simulink model "idealvehicle"  (R2020b)
settings: Solver=ode4  StartTime=0  StopTime=endtime  FixedStep=0.1  MaxStep=0.05  RelTol=1e-5
values from neighbouring files (symbols this model uses):
  Av = 2.55    [InitiateIDEAL.m]
  Cd = 0.79    [InitiateIDEAL.m]
  Cr = 0.00576    [InitiateIDEAL.m]
  Density = (85*19.6e6 + 15*32e6)/100    (= 21460000)    [InitiateIDEAL.m]
  grav = 9.81    [InitiateIDEAL.m]
  Mv = 40000    [InitiateIDEAL.m]
  Pmax = 450000    [InitiateIDEAL.m]
  rho_air = 1.2    [InitiateIDEAL.m]
  rw = 0.506    [InitiateIDEAL.m]
settings Model: ExtModeTrigMode=oneshot  ExtModeArmWhenConnect=off  Creator=Mats  LastModifiedBy=ielmats
settings DataIOCC: SaveFormat=Array  SignalLoggingSaveFormat=ModelDataLogs  ReturnWorkspaceOutputs=off  SignalLoggingName=sigsOut
settings OptimizationCC: BlockReduction=off  BooleanDataType=off  ExpressionDepthLimit=2147483647  InitFltsAndDblsToZero=on  LifeSpan=inf
settings DebuggingCC: ConsistencyChecking=warning  SaveWithParameterizedLinksMsg=none  UnderspecifiedInitializationDetection=Classic  MergeDetectMultiDrivingBlocksExec=none  SignalResolutionControl=TryResolveAllWithWarning  MultiTaskDSMMsg=warning  MultiTaskCondExecSysMsg=none  UnnecessaryDatatypeConvMsg=warning  UnconnectedInputMsg=none  UnconnectedOutputMsg=none  UnconnectedLineMsg=none  StateNameClashWarn=warning  SFUnexpectedBacktrackingDiag=warning  SFNoUnconditionalDefaultTransitionDiag=warning  ArithmeticOperatorsInVariantConditions=warning
settings HardwareCC: ProdBitPerPointer=32  ProdBitPerSizeT=32  ProdBitPerPtrDiffT=32  ProdLargestAtomicFloat=None  ProdIntDivRoundTo=Undefined  ProdEndianess=Unspecified  ProdWordSize=32  ProdHWDeviceType=32-bit Generic  TargetUnknown=on
settings ModelReferenceCC: PropagateSignalLabelsOutOfModel=off
settings SFSimCC: SimUseLocalCustomCode=off  CustomCodeUndefinedFunction=UseInterfaceOnly
settings RTWCC: RTWUseLocalCustomCode=off
settings CodeAppCC: StateflowObjectComments=on
settings GRTTargetCC: TargetLangStandard=C89/C90 (ANSI)  CombineOutputUpdateFcns=off  GRTInterface=on
settings ConfigComp: CovMetricSettings=dw  CovSaveCumulativeToWorkspaceVar=on  CovSaveSingleToWorkspaceVar=on  CovExternalEMLEnable=off

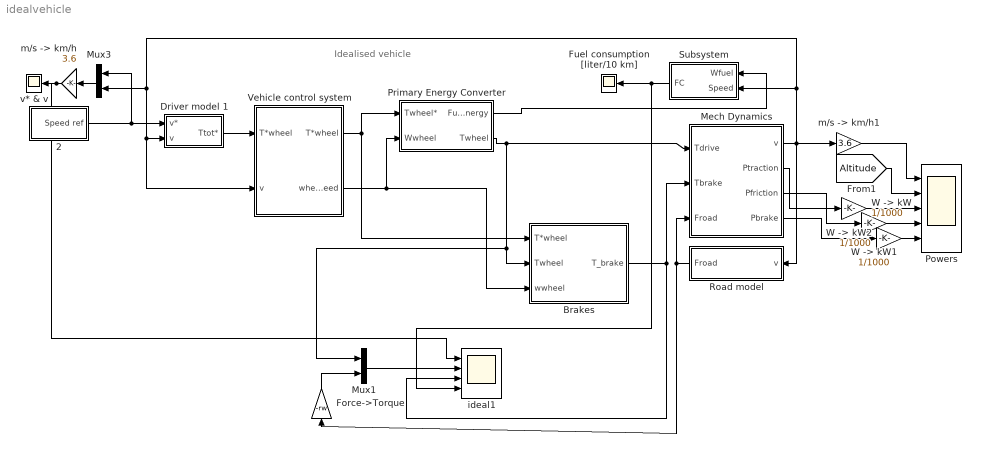
== system idealvehicle ==
  note: Idealised vehicle
  " 2" : Subsystem
  Brakes : Subsystem
  Driver model 1 : Subsystem  mask{Mv=Mv, rw=rw, Pmax=Pmax}
      mask prompts: Mv "Vehicle Mass"; rw "Wheel Radius"; Pmax "Max Wheel Power"
      mask init:
      | Ti = 2 + 1*(Mv-1000)/19000;
      | Kv=4*Mv/Ti;
  Force->Torque : Gain  Gain=-rw  SaturateOnIntegerOverflow=on  OutDataTypeStr=Inherit: Same as input  ParamDataTypeStr=Inherit: Same as input
  Fuel consumption [liter/10 km] : Scope
  Mech Dynamics : Subsystem
  Mux1 : Mux  Inputs=2
  Mux3 : Mux  Inputs=2
  Powers : Scope  NumInputPorts=5
  Primary Energy Converter : Subsystem
  Road model : Subsystem
  Subsystem : Subsystem
  Vehicle control system : Subsystem
  "W -> kW" : Gain  Gain=1/1000  SaturateOnIntegerOverflow=on  OutDataTypeStr=Inherit: Same as input  ParamDataTypeStr=Inherit: Same as input
  "W -> kW1" : Gain  Gain=1/1000  SaturateOnIntegerOverflow=on  OutDataTypeStr=Inherit: Same as input  ParamDataTypeStr=Inherit: Same as input
  "W -> kW2" : Gain  Gain=1/1000  SaturateOnIntegerOverflow=on  OutDataTypeStr=Inherit: Same as input  ParamDataTypeStr=Inherit: Same as input
  ideal1 : Scope  NumInputPorts=4
  "m/s -> km/h" : Gain  Gain=3.6  SaturateOnIntegerOverflow=on  OutDataTypeStr=Inherit: Same as input  ParamDataTypeStr=Inherit: Same as input
  "m/s -> km/h1" : Gain  Gain=3.6  SaturateOnIntegerOverflow=on  OutDataTypeStr=Inherit: Same as input  ParamDataTypeStr=Inherit: Same as input
  v* & v : Scope
  wires:
  Primary Energy Converter/2(Twheel) -> Brakes/2(Twheel), Mux1/1, Mech Dynamics/1(Tdrive)
  " 2"/1(Speed ref) -> Mux3/1, Driver model 1/1(v*)
  Driver model 1/1(Ttot*) -> Vehicle control system/1(T*wheel)
  Mux3/1 -> "m/s -> km/h"/1
  Vehicle control system/1("T*wheel ") -> Primary Energy Converter/1(Twheel*), Brakes/1(T*wheel)
  Mech Dynamics/1(v) -> Road model/1("v "), Subsystem/2(Speed), Driver model 1/2(v), Vehicle control system/2(v), Mux3/2, "m/s -> km/h1"/1
  Road model/1(Froad) -> Force->Torque/1, Mech Dynamics/3(Froad)
  Brakes/1(T_brake) -> ideal1/3, Mech Dynamics/2(Tbrake)
  Primary Energy Converter/1(Fuel energy) -> Subsystem/1(Wfuel)
  "m/s -> km/h"/1 -> ideal1/1, v* & v/1
  Subsystem/1(FC) -> Fuel consumption [liter/10 km]/1, ideal1/4
  Vehicle control system/2(wheel speed) -> Primary Energy Converter/2(Wwheel), Brakes/3(wwheel)
  Mux1/1 -> ideal1/2
  Force->Torque/1 -> Mux1/2
  [Altitude] -> Powers/2
  Mech Dynamics/3(Pfriction) -> "W -> kW1"/1
  Mech Dynamics/4(Pbrake) -> "W -> kW2"/1
  "m/s -> km/h1"/1 -> Powers/1
  Mech Dynamics/2(Ptraction) -> "W -> kW"/1
  "W -> kW"/1 -> Powers/3
  "W -> kW1"/1 -> Powers/4
  "W -> kW2"/1 -> Powers/5

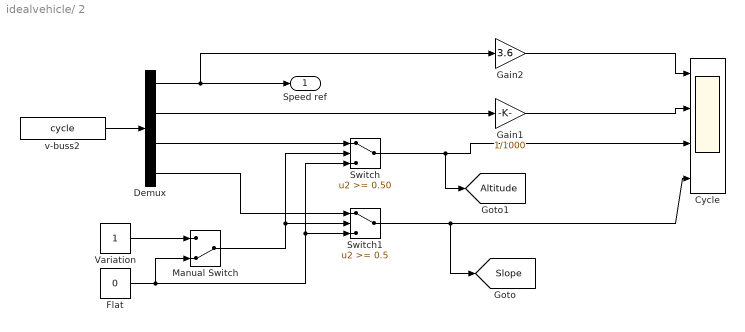
== system idealvehicle/ 2 ==
  Cycle : Scope  NumInputPorts=4
  Demux : Demux
  Flat : Constant  Value=0
  Gain1 : Gain  Gain=1/1000  SaturateOnIntegerOverflow=on  OutDataTypeStr=Inherit: Same as input  ParamDataTypeStr=Inherit: Same as input
  Gain2 : Gain  Gain=3.6  SaturateOnIntegerOverflow=on  OutDataTypeStr=Inherit: Same as input  ParamDataTypeStr=Inherit: Same as input
  Manual Switch : ManualSwitch  CurrentSetting=0
  Switch : Switch  Threshold=0.50
  Switch1 : Switch  Threshold=0.5
  Variation : Constant
  v-buss2 : FromWorkspace  VariableName=cycle  SampleTime=.2  ZeroCross=off
  Speed ref : Outport  VectorParamsAs1DForOutWhenUnconnected=off
  tag scope: Altitude=global, Slope=global
  wires:
  v-buss2/1 -> Demux/1
  Demux/4 -> Switch1/1
  Demux/1 -> Speed ref/1, Gain2/1
  Demux/3 -> Switch/1
  Demux/2 -> Gain1/1
  Flat/1 -> Switch1/3, Switch/3, Manual Switch/2
  Switch/1 -> Cycle/3, [Altitude]
  Switch1/1 -> Cycle/4, [Slope]
  Variation/1 -> Manual Switch/1
  Manual Switch/1 -> Switch/2, Switch1/2
  Gain1/1 -> Cycle/2
  Gain2/1 -> Cycle/1

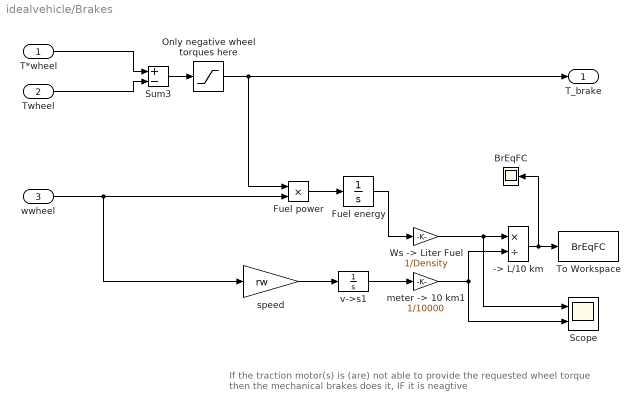
== system idealvehicle/Brakes ==
  note: If the traction motor(s) is (are) not able to provide the requested wheel torque
      | then the mechanical brakes does it, IF it is neagtive
  T*wheel : Inport
  Twheel : Inport  Port=2
  wwheel : Inport  Port=3
  -> L/10 km : Product  Inputs=*/  InputSameDT=on  SaturateOnIntegerOverflow=on  OutDataTypeStr=Inherit: Same as first input
  BrEqFC : Scope
  "Fuel energy " : Integrator
  Fuel power : Product  Inputs=**  InputSameDT=on  SaturateOnIntegerOverflow=on  OutDataTypeStr=Inherit: Same as first input
  Only negative wheel torques here : Saturate  UpperLimit=0  LowerLimit=-inf
  Scope : Scope  NumInputPorts=2
  Sum3 : Sum  Inputs=+-  InputSameDT=on  SaturateOnIntegerOverflow=on  OutDataTypeStr=Inherit: Same as first input
  To Workspace : ToWorkspace  VariableName=BrEqFC  SampleTime=-1
  "Ws -> Liter Fuel" : Gain  Gain=1/Density  SaturateOnIntegerOverflow=on  OutDataTypeStr=Inherit: Same as input  ParamDataTypeStr=Inherit: Same as input
  "meter -> 10 km1" : Gain  Gain=1/10000  SaturateOnIntegerOverflow=on  OutDataTypeStr=Inherit: Same as input  ParamDataTypeStr=Inherit: Same as input
  speed : Gain  Gain=rw  SaturateOnIntegerOverflow=on  OutDataTypeStr=Inherit: Same as input  ParamDataTypeStr=Inherit: Same as input
  v->s1 : Integrator  InitialCondition=100  LimitOutput=on  LowerSaturationLimit=100
  T_brake : Outport  InitialOutput=0  VectorParamsAs1DForOutWhenUnconnected=off
  wires:
  Sum3/1 -> Only negative wheel torques here/1
  T*wheel/1 -> Sum3/1
  Twheel/1 -> Sum3/2
  Only negative wheel torques here/1 -> T_brake/1, Fuel power/1
  wwheel/1 -> speed/1, Fuel power/2
  v->s1/1 -> "meter -> 10 km1"/1
  speed/1 -> v->s1/1
  "Fuel energy "/1 -> "Ws -> Liter Fuel"/1
  Fuel power/1 -> "Fuel energy "/1
  "Ws -> Liter Fuel"/1 -> -> L/10 km/1, Scope/1
  "meter -> 10 km1"/1 -> -> L/10 km/2, Scope/2
  -> L/10 km/1 -> To Workspace/1, BrEqFC/1

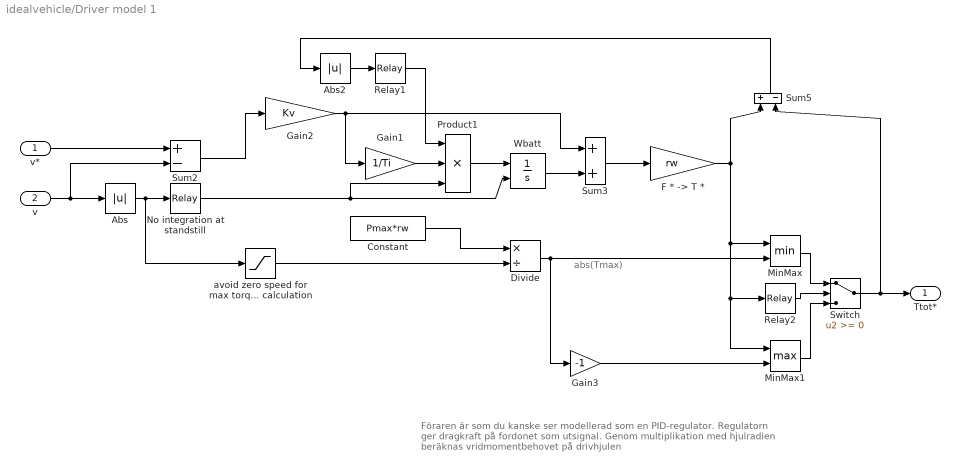
== system idealvehicle/Driver model 1 ==
  note: Föraren är som du kanske ser modellerad som en PID-regulator.
      | Regulatorn ger dragkraft på fordonet som utsignal. Genom
      | multiplikation med hjulradien beräknas vridmomentbehovet på drivhjulen
  note: abs(Tmax)
  v* : Inport
  v : Inport  Port=2
  Abs : Abs  SaturateOnIntegerOverflow=on
  Abs2 : Abs  SaturateOnIntegerOverflow=on
  Constant : Constant  Value=Pmax*rw
  Divide : Product  Inputs=*/
  "F * -> T *" : Gain  Gain=rw  SaturateOnIntegerOverflow=on  OutDataTypeStr=Inherit: Same as input  ParamDataTypeStr=Inherit: Same as input
  Gain1 : Gain  Gain=1/Ti  SaturateOnIntegerOverflow=on  OutDataTypeStr=Inherit: Same as input  ParamDataTypeStr=Inherit: Same as input
  Gain2 : Gain  Gain=Kv  SaturateOnIntegerOverflow=on  OutDataTypeStr=Inherit: Same as input  ParamDataTypeStr=Inherit: Same as input
  Gain3 : Gain  Gain=-1  SaturateOnIntegerOverflow=on  OutDataTypeStr=Inherit: Same as input  ParamDataTypeStr=Inherit: Same as input
  MinMax : MinMax  Inputs=2
  MinMax1 : MinMax  Function=max  Inputs=2
  No integration at standstill : Relay  OnSwitchValue=0.3  OffSwitchValue=0.3-eps
  Product1 : Product  Inputs=3  InputSameDT=on  SaturateOnIntegerOverflow=on  OutDataTypeStr=Inherit: Same as first input
  Relay1 : Relay  OnOutputValue=0  OffOutputValue=1
  Relay2 : Relay  OnOutputValue=10  OffOutputValue=1
  Sum2 : Sum  Inputs=+-  InputSameDT=on  SaturateOnIntegerOverflow=on  OutDataTypeStr=Inherit: Same as first input
  Sum3 : Sum  InputSameDT=on  SaturateOnIntegerOverflow=on  OutDataTypeStr=Inherit: Same as first input
  Sum5 : Sum  Inputs=+-  InputSameDT=on  SaturateOnIntegerOverflow=on  OutDataTypeStr=Inherit: Same as first input
  Switch : Switch
  Wbatt : Integrator  ExternalReset=falling  LimitOutput=on  UpperSaturationLimit=1000  LowerSaturationLimit=-10000
  avoid zero speed for max torque calculation : Saturate  UpperLimit=inf  LowerLimit=5/3.6
  Ttot* : Outport  InitialOutput=0  VectorParamsAs1DForOutWhenUnconnected=off
  wires:
  Sum5/1 -> Abs2/1
  Relay1/1 -> Product1/1
  Abs2/1 -> Relay1/1
  Gain1/1 -> Product1/2
  Abs/1 -> No integration at standstill/1, avoid zero speed for max torque calculation/1
  Product1/1 -> Wbatt/1
  Sum3/1 -> "F * -> T *"/1
  Wbatt/1 -> Sum3/2
  "F * -> T *"/1 -> Sum5/1, MinMax/1, MinMax1/1, Relay2/1
  Gain2/1 -> Gain1/1, Sum3/1
  No integration at standstill/1 -> Product1/3, Wbatt/2
  Sum2/1 -> Gain2/1
  v*/1 -> Sum2/1
  v/1 -> Abs/1, Sum2/2
  Constant/1 -> Divide/1
  avoid zero speed for max torque calculation/1 -> Divide/2
  Divide/1 -> Gain3/1, MinMax/2
  Gain3/1 -> MinMax1/2
  Relay2/1 -> Switch/2
  MinMax/1 -> Switch/1
  MinMax1/1 -> Switch/3
  Switch/1 -> Ttot*/1, Sum5/2

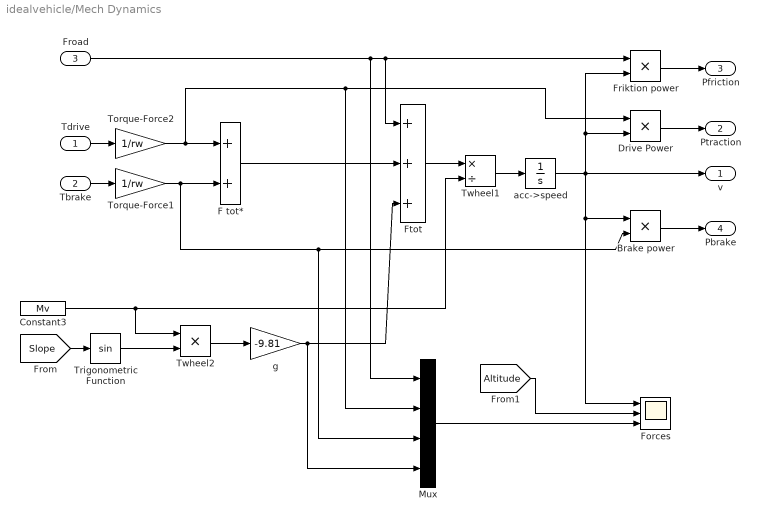
== system idealvehicle/Mech Dynamics ==
  Tdrive : Inport
  Tbrake : Inport  Port=2
  Froad : Inport  Port=3
  Brake power : Product  InputSameDT=on  SaturateOnIntegerOverflow=on  OutDataTypeStr=Inherit: Same as first input
  Constant3 : Constant  Value=Mv
  Drive Power : Product  InputSameDT=on  SaturateOnIntegerOverflow=on  OutDataTypeStr=Inherit: Same as first input
  F tot* : Sum  InputSameDT=on  SaturateOnIntegerOverflow=on  OutDataTypeStr=Inherit: Same as first input
  Forces : Scope  NumInputPorts=3
  Friktion power : Product  InputSameDT=on  SaturateOnIntegerOverflow=on  OutDataTypeStr=Inherit: Same as first input
  Ftot : Sum  Inputs=+++  InputSameDT=on  SaturateOnIntegerOverflow=on  OutDataTypeStr=Inherit: Same as first input
  Mux : Mux
  Torque-Force1 : Gain  Gain=1/rw  SaturateOnIntegerOverflow=on  OutDataTypeStr=Inherit: Same as input  ParamDataTypeStr=Inherit: Same as input
  Torque-Force2 : Gain  Gain=1/rw  SaturateOnIntegerOverflow=on  OutDataTypeStr=Inherit: Same as input  ParamDataTypeStr=Inherit: Same as input
  Trigonometric Function : Trigonometry
  Twheel1 : Product  Inputs=*/  InputSameDT=on  SaturateOnIntegerOverflow=on  OutDataTypeStr=Inherit: Same as first input
  Twheel2 : Product  Inputs=**  InputSameDT=on  SaturateOnIntegerOverflow=on  OutDataTypeStr=Inherit: Same as first input
  acc->speed : Integrator  LimitOutput=on  LowerSaturationLimit=0
  g : Gain  Gain=-9.81  SaturateOnIntegerOverflow=on  OutDataTypeStr=Inherit: Same as input  ParamDataTypeStr=Inherit: Same as input
  v : Outport  InitialOutput=0  VectorParamsAs1DForOutWhenUnconnected=off
  Ptraction : Outport  Port=2  InitialOutput=0  VectorParamsAs1DForOutWhenUnconnected=off
  Pfriction : Outport  Port=3  InitialOutput=0  VectorParamsAs1DForOutWhenUnconnected=off
  Pbrake : Outport  Port=4  InitialOutput=0  VectorParamsAs1DForOutWhenUnconnected=off
  wires:
  Twheel1/1 -> acc->speed/1
  Tdrive/1 -> Torque-Force2/1
  acc->speed/1 -> Friktion power/2, Drive Power/2, Brake power/1, Forces/1, v/1
  Tbrake/1 -> Torque-Force1/1
  F tot*/1 -> Ftot/2
  Ftot/1 -> Twheel1/1
  Froad/1 -> Ftot/1, Friktion power/1, Mux/1
  Friktion power/1 -> Pfriction/1
  Constant3/1 -> Twheel1/2, Twheel2/1
  Trigonometric Function/1 -> Twheel2/2
  Twheel2/1 -> g/1
  g/1 -> Mux/4, Ftot/3
  [Slope] -> Trigonometric Function/1
  [Altitude] -> Forces/2
  Mux/1 -> Forces/3
  Drive Power/1 -> Ptraction/1
  Torque-Force1/1 -> F tot*/2, Mux/3, Brake power/2
  Torque-Force2/1 -> F tot*/1, Drive Power/1, Mux/2
  Brake power/1 -> Pbrake/1

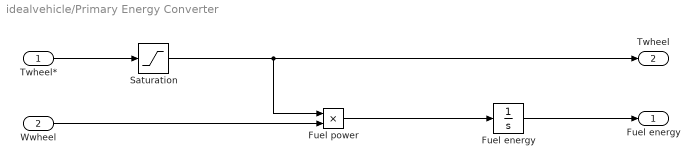
== system idealvehicle/Primary Energy Converter ==
  Twheel* : Inport
  Wwheel : Inport  Port=2
  "Fuel energy " : Integrator
  Fuel power : Product  Inputs=**  InputSameDT=on  SaturateOnIntegerOverflow=on  OutDataTypeStr=Inherit: Same as first input
  Saturation : Saturate  UpperLimit=inf  LowerLimit=0
  Fuel energy : Outport  InitialOutput=0  VectorParamsAs1DForOutWhenUnconnected=off
  Twheel : Outport  Port=2  InitialOutput=0  VectorParamsAs1DForOutWhenUnconnected=off
  wires:
  "Fuel energy "/1 -> Fuel energy/1
  Twheel*/1 -> Saturation/1
  Wwheel/1 -> Fuel power/2
  Fuel power/1 -> "Fuel energy "/1
  Saturation/1 -> Twheel/1, Fuel power/1

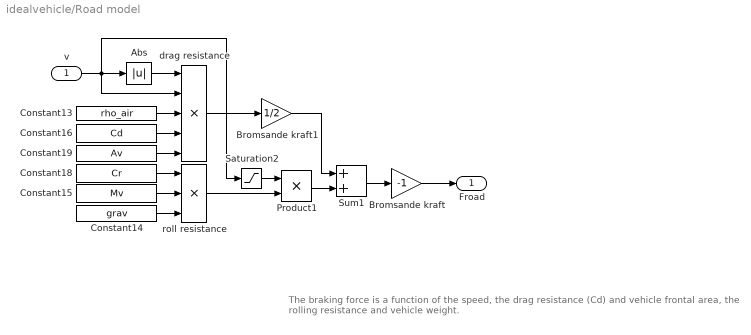
== system idealvehicle/Road model ==
  note: The braking force is  a function  of the speed, the drag resistance (Cd) and vehicle frontal area,
      | the rolling resistance and vehicle weight.
  "v " : Inport
  Abs : Abs  SaturateOnIntegerOverflow=on
  Bromsande kraft : Gain  Gain=-1  SaturateOnIntegerOverflow=on  OutDataTypeStr=Inherit: Same as input  ParamDataTypeStr=Inherit: Same as input
  Bromsande kraft1 : Gain  Gain=1/2  SaturateOnIntegerOverflow=on  OutDataTypeStr=Inherit: Same as input  ParamDataTypeStr=Inherit: Same as input
  Constant13 : Constant  Value=rho_air
  Constant14 : Constant  Value=grav
  Constant15 : Constant  Value=Mv
  Constant16 : Constant  Value=Cd
  Constant18 : Constant  Value=Cr
  Constant19 : Constant  Value=Av
  Product1 : Product  InputSameDT=on  SaturateOnIntegerOverflow=on  OutDataTypeStr=Inherit: Same as first input
  Saturation2 : Saturate  UpperLimit=1  LowerLimit=-1
  Sum1 : Sum  InputSameDT=on  SaturateOnIntegerOverflow=on  OutDataTypeStr=Inherit: Same as first input
  drag resistance : Product  Inputs=5  InputSameDT=on  SaturateOnIntegerOverflow=on  OutDataTypeStr=Inherit: Same as first input
  roll resistance : Product  Inputs=3  InputSameDT=on  SaturateOnIntegerOverflow=on  OutDataTypeStr=Inherit: Same as first input
  Froad : Outport  InitialOutput=0  VectorParamsAs1DForOutWhenUnconnected=off
  wires:
  Abs/1 -> drag resistance/1
  Constant15/1 -> roll resistance/2
  Constant18/1 -> roll resistance/1
  Constant19/1 -> drag resistance/5
  Constant16/1 -> drag resistance/4
  Constant13/1 -> drag resistance/3
  Constant14/1 -> roll resistance/3
  Product1/1 -> Sum1/2
  drag resistance/1 -> Bromsande kraft1/1
  Saturation2/1 -> Product1/1
  roll resistance/1 -> Product1/2
  Sum1/1 -> Bromsande kraft/1
  "v "/1 -> Abs/1, Saturation2/1, drag resistance/2
  Bromsande kraft/1 -> Froad/1
  Bromsande kraft1/1 -> Sum1/1

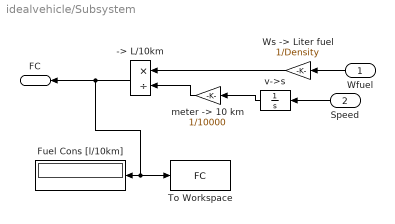
== system idealvehicle/Subsystem ==
  Wfuel : Inport
  Speed : Inport  Port=2
  -> L/10km : Product  Inputs=*/  InputSameDT=on  SaturateOnIntegerOverflow=on  OutDataTypeStr=Inherit: Same as first input
  Fuel Cons [l/10km] : Display
  To Workspace : ToWorkspace  VariableName=FC  SampleTime=-1
  "Ws -> Liter fuel" : Gain  Gain=1/Density  SaturateOnIntegerOverflow=on  OutDataTypeStr=Inherit: Same as input  ParamDataTypeStr=Inherit: Same as input
  "meter -> 10 km" : Gain  Gain=1/10000  SaturateOnIntegerOverflow=on  OutDataTypeStr=Inherit: Same as input  ParamDataTypeStr=Inherit: Same as input
  v->s : Integrator  InitialCondition=100  LimitOutput=on  LowerSaturationLimit=100
  FC : Outport  VectorParamsAs1DForOutWhenUnconnected=off
  wires:
  "Ws -> Liter fuel"/1 -> -> L/10km/1
  v->s/1 -> "meter -> 10 km"/1
  -> L/10km/1 -> FC/1, Fuel Cons [l/10km]/1, To Workspace/1
  Wfuel/1 -> "Ws -> Liter fuel"/1
  Speed/1 -> v->s/1
  "meter -> 10 km"/1 -> -> L/10km/2

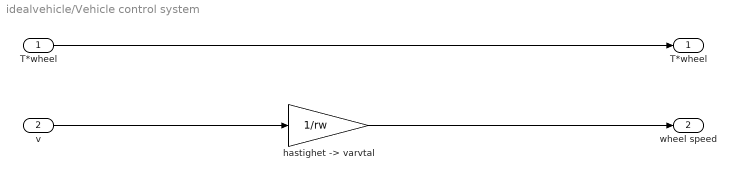
== system idealvehicle/Vehicle control system ==
  T*wheel : Inport
  v : Inport  Port=2
  "hastighet -> varvtal" : Gain  Gain=1/rw  SaturateOnIntegerOverflow=on  OutDataTypeStr=Inherit: Same as input  ParamDataTypeStr=Inherit: Same as input
  "T*wheel " : Outport  VectorParamsAs1DForOutWhenUnconnected=off
  wheel speed : Outport  Port=2  VectorParamsAs1DForOutWhenUnconnected=off
  wires:
  T*wheel/1 -> "T*wheel "/1
  v/1 -> "hastighet -> varvtal"/1
  "hastighet -> varvtal"/1 -> wheel speed/1
